simulink model "fw_pos_control"  (R2021a)
settings: Solver=FixedStepAuto  StartTime=0.0  StopTime=5  FixedStep=0.02  RelTol=1e-3
undefined symbols (not defined in the file): DiscIntNeverNeededParam, DT_DEFAULT, FW_AIRSPD_MAX, FW_AIRSPD_MIN, FW_L1_DAMPING, FW_L1_PERIOD, FW_L1_R_SLEW_MAX, FW_R_LIM, FW_T_CLMB_MAX, FW_T_HRATE_FF, FW_T_I_GAIN_PIT, FW_T_I_GAIN_THR, FW_T_PTCH_DAMP, FW_T_RLL2THR, FW_T_SEB_R_FF, FW_T_SINK_MAX, FW_T_SINK_MIN, FW_T_SPD_OMEGA, FW_T_STE_R_TC, FW_T_TAS_TC, FW_T_THR_DAMP, FW_T_VERT_ACC, FW_THR_CRUISE, FW_THR_MAX, FW_THR_MIN, FW_THR_SLEW_MAX, GRAVITY, magnitude
libraries: simulink x28, vrlib x3
(part 2 of 4)

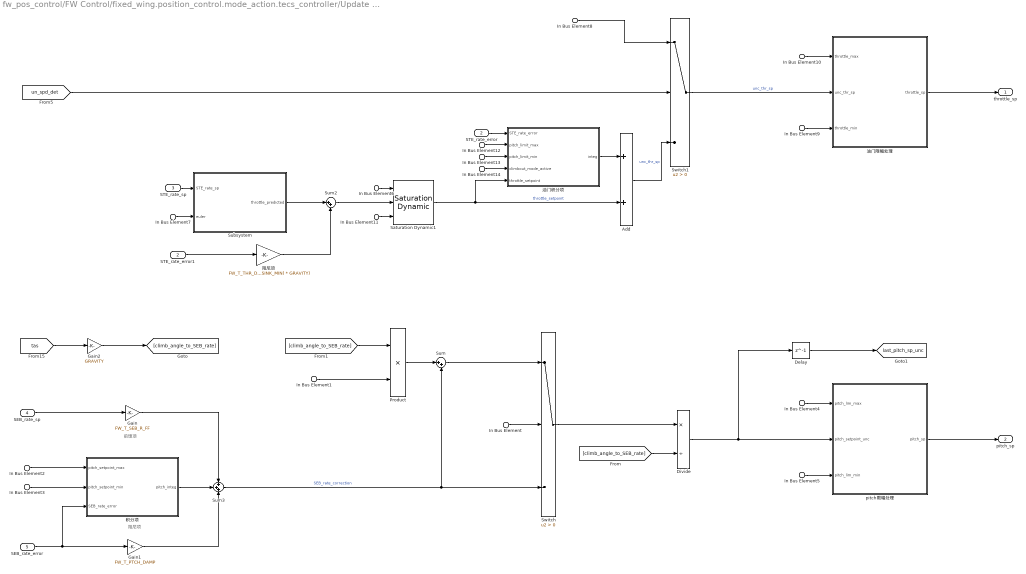
== system fw_pos_control/FW Control/fixed_wing.position_control.mode_action.tecs_controller/Update Throttle Setpoint and Pitch Setpoint ==
  note: 前馈项
  note: 阻尼项
  In Bus Element : Inport  PortName=tecs  Element=climb_out_setpoint
  In Bus Element14 : Inport  PortName=tecs  Element=climb_out_setpoint
  In Bus Element2 : Inport  PortName=tecs  Element=pitch_limit_max
  In Bus Element4 : Inport  PortName=tecs  Element=pitch_limit_max
  In Bus Element12 : Inport  PortName=tecs  Element=pitch_limit_max
  In Bus Element{1,3,5,13} (4 alike) : Inport  PortName=tecs  Element=pitch_limit_min
  In Bus Element11 : Inport  PortName=tecs  Element=throttle_min
  In Bus Element9 : Inport  PortName=tecs  Element=throttle_min
  In Bus Element10 : Inport  PortName=tecs  Element=throttle_max
  In Bus Element8 : Inport  PortName=tecs  Element=throttle_max
  In Bus Element6 : Inport  PortName=tecs  Element=throttle_max
  In Bus Element7 : Inport  PortName=tecs  Element=euler
  STE_rate_error : Inport  Port=2
  STE_rate_sp : Inport  Port=3
  SEB_rate_sp : Inport  Port=4
  SEB_rate_error : Inport  Port=5
  Add : Sum
  Delay : Delay  DelayLength=1
  Divide : Product  Inputs=*/
  Gain : Gain  Gain=FW_T_SEB_R_FF
      settings: AttributesFormatString=%<Gain>
  Gain1 : Gain  Gain=FW_T_PTCH_DAMP
      settings: AttributesFormatString=%<Gain>
  Gain2 : Gain  Gain=GRAVITY
      settings: AttributesFormatString=%<Gain>
  Product : Product
  STE_rate_error1 : InportShadow  Port=2
  Saturation Dynamic1 : simulink/Discontinuities/Saturation Dynamic  OutMin=[]  OutMax=[]  OutDataTypeStr=Inherit: Same as second input  OutDataType=fixdt(1, 16)  OutScaling=2^-10  DoSatur=off
  Subsystem : Subsystem
  Sum : Sum  Inputs=|++
  Sum2 : Sum  Inputs=|++
  Sum3 : Sum  Inputs=+++
  Switch : Switch  Criteria=u2 > Threshold
  Switch1 : Switch  Criteria=u2 > Threshold
  pitch限幅处理 : Subsystem
  油门积分项 : Subsystem
  油门限幅处理 : Subsystem
  积分项 : Subsystem
  阻尼项 : Gain  Gain=FW_T_THR_DAMP / ((FW_T_CLMB_MAX - FW_T_SINK_MIN) * GRAVITY)  OutDataTypeStr=single
      settings: AttributesFormatString=%<Gain>
  throttle_sp : Outport
  pitch_sp : Outport  Port=2
  tag scope: last_pitch_sp_unc=global
  wires:
  pitch限幅处理/1(pitch_sp) -> pitch_sp/1
  Divide/1 -> Delay/1, pitch限幅处理/2(pitch_setpoint_unc)
  SEB_rate_error/1 -> 积分项/3(SEB_rate_error), Gain1/1
  Delay/1 -> [last_pitch_sp_unc]
  积分项/1(pitch_integ) -> Sum3/2
  Gain/1 -> Sum3/1
  SEB_rate_sp/1 -> Gain/1
  Gain1/1 -> Sum3/3
  Sum3/1 -> Sum/2, Switch/3  "SEB_rate_correction"
  In Bus Element/1 -> Switch/2
  In Bus Element3/1 -> 积分项/2(pitch_setpoint_min)
  In Bus Element2/1 -> 积分项/1(pitch_setpoint_max)
  Switch/1 -> Divide/1
  Gain2/1 -> [climb_angle_to_SEB_rate]
  [tas] -> Gain2/1
  [climb_angle_to_SEB_rate] -> Divide/2
  [climb_angle_to_SEB_rate] -> Product/1
  In Bus Element1/1 -> Product/2
  Product/1 -> Sum/1
  Sum/1 -> Switch/1
  In Bus Element4/1 -> pitch限幅处理/1(pitch_lim_max)
  In Bus Element5/1 -> pitch限幅处理/3(pitch_lim_min)
  Saturation Dynamic1/1 -> 油门积分项/5(throttle_setpoint), Add/2  "throttle_setpoint"
  Subsystem/1(throttle_predicted) -> Sum2/1
  Switch1/1 -> 油门限幅处理/2(unc_thr_sp)  "unc_thr_sp"
  In Bus Element9/1 -> 油门限幅处理/3(throttle_min)
  Add/1 -> Switch1/3  "unc_thr_sp"
  In Bus Element6/1 -> Saturation Dynamic1/1
  In Bus Element8/1 -> Switch1/1
  阻尼项/1 -> Sum2/2
  [un_spd_det] -> Switch1/2
  In Bus Element10/1 -> 油门限幅处理/1(throttle_max)
  油门限幅处理/1(throttle_sp) -> throttle_sp/1
  STE_rate_error/1 -> 油门积分项/1(STE_rate_error)
  In Bus Element11/1 -> Saturation Dynamic1/3
  油门积分项/1(integ) -> Add/1
  Sum2/1 -> Saturation Dynamic1/2
  STE_rate_sp/1 -> Subsystem/1(STE_rate_sp)
  In Bus Element12/1 -> 油门积分项/2(pitch_limit_max)
  In Bus Element14/1 -> 油门积分项/4(climbout_mode_active)
  In Bus Element13/1 -> 油门积分项/3(pitch_limit_min)
  In Bus Element7/1 -> Subsystem/2(euler)
  STE_rate_error1/1 -> 阻尼项/1

== system fw_pos_control/FW Control/fixed_wing.position_control.mode_action.l1_navigate_loiter/Circle Mode/PD Terms ==
  note: $lateral\_accel\_sp\_circle\_pd = (xtrack\_err\_circle \times K\_crosstrack + xtrack\_vel\_circle \times K\_velocity);$
  xtrack_err_circle : Inport
  xtrack_vel_circle : Inport  Port=2
  circle_mode : Inport  Port=3
  AND : Logic  IconShape=distinctive  AllPortsSameDT=off  OutDataTypeStr=boolean
  Compare To Zero : simulink/Logic and Bit Operations/Compare To Zero  relop=<  OutDataTypeStr=boolean
  Gain1 : Gain  Gain=(2 * pi / FW_L1_PERIOD)^2
      settings: AttributesFormatString=%<Gain>
  Gain2 : Gain  Gain=(2 * pi / FW_L1_PERIOD)^2
      settings: AttributesFormatString=%<Gain>
  Gain3 : Gain  Gain=2 * FW_L1_DAMPING * (2 * pi / FW_L1_PERIOD)
      settings: AttributesFormatString=%<Gain>
  Gain5 : Gain  Gain=2 * FW_L1_DAMPING * (2 * pi / FW_L1_PERIOD)
      settings: AttributesFormatString=%<Gain>
  Saturation2 : Saturate  UpperLimit=0  LowerLimit=-inf
      settings: AttributesFormatString=[%<LowerLimit>,%<UpperLimit>]
  Sum1 : Sum  Inputs=|++
  Sum4 : Sum  Inputs=|++
  Switch2 : Switch  Criteria=u2 > Threshold
  xtrack_err_circle_1 : InportShadow
  xtrack_vel_circle_1 : InportShadow  Port=2
  lateral_accel_sp_circle_pd : Outport
  wires:
  xtrack_vel_circle_1/1 -> Gain5/1
  Saturation2/1 -> Switch2/1
  circle_mode/1 -> AND/2
  [tangent_vel] -> Compare To Zero/1
  Gain5/1 -> Sum4/2
  xtrack_err_circle/1 -> Gain2/1
  Compare To Zero/1 -> AND/1
  Gain1/1 -> Sum4/1
  Sum4/1 -> Switch2/3
  Gain3/1 -> Sum1/2
  xtrack_vel_circle/1 -> Gain3/1
  Sum1/1 -> Saturation2/1
  xtrack_err_circle_1/1 -> Gain1/1
  AND/1 -> Switch2/2
  Gain2/1 -> Sum1/1
  Switch2/1 -> lateral_accel_sp_circle_pd/1

== system fw_pos_control/FW Control/fixed_wing.position_control.mode_action.l1_navigate_loiter/Switch Lateral Accel Setpoint/If Action Subsystem ==
  lateral_accel_sp_center : Inport
  Action Port : ActionPort  ActionPortLabel=if(u1)
  Constant : Constant  Value=false
  circle_mode : Outport
  lateral_accel_sp : Outport  Port=2
  wires:
  Constant/1 -> circle_mode/1
  lateral_accel_sp_center/1 -> lateral_accel_sp/1

== system fw_pos_control/FW Control/fixed_wing.position_control.mode_action.l1_navigate_loiter/Switch Lateral Accel Setpoint/If Action Subsystem1 ==
  lateral_accel_sp_circle1 : Inport
  Action Port : ActionPort  ActionPortLabel=else
  Constant1 : Constant  Value=true
  lateral_accel_sp : Outport
  circle_mode : Outport  Port=2
  wires:
  lateral_accel_sp_circle1/1 -> lateral_accel_sp/1
  Constant1/1 -> circle_mode/1

== system fw_pos_control/FW Control/fixed_wing.position_control.mode_action.l1_navigate_loiter/Switch Lateral Accel Setpoint/Update Roll Setpoint ==
  att_sp_roll_body : Inport  PortDimensions=1
  lateral_accel : Inport  Port=2
  Compare To Zero : simulink/Logic and Bit Operations/Compare To Zero  relop=>  OutDataTypeStr=boolean
  Constant1 : Constant  Value=FW_L1_R_SLEW_MAX
      settings: AttributesFormatString=%<Value>
  Constant2 : Constant  Value=FW_L1_R_SLEW_MAX
      settings: AttributesFormatString=%<Value>
  Gain : Gain  Gain=1.0 / GRAVITY
      settings: AttributesFormatString=%<Gain>
  IsFinite1 : RelationalOperator  Operator=isFinite  OutDataTypeStr=boolean  RndMeth=Simplest
  Saturation : Saturate  UpperLimit=FW_R_LIM  LowerLimit=-FW_R_LIM
      settings: AttributesFormatString=[%<LowerLimit>,%<UpperLimit>]
  Saturation Dynamic : simulink/Discontinuities/Saturation Dynamic  OutMin=[]  OutMax=[]  OutDataTypeStr=Inherit: Same as second input  OutDataType=fixdt(1, 16)  OutScaling=2^-10  DoSatur=off
  Sum : Sum  Inputs=|++
  Sum1 : Sum  Inputs=-+|
  Switch1 : Switch  Criteria=u2 > Threshold
  Switch2 : Switch  Criteria=u2 > Threshold
  Weighted Sample Time : SampleTimeMath  TsampMathOp=*
  att_sp_roll_body_1 : InportShadow  PortDimensions=1
  att_sp_roll_body_2 : InportShadow  PortDimensions=1
  roll_sp : Outport
  wires:
  att_sp_roll_body/1 -> Sum/1
  Sum/1 -> Saturation Dynamic/1
  Weighted Sample Time/1 -> Sum/2, Sum1/1
  att_sp_roll_body_2/1 -> Switch2/3
  Saturation/1 -> IsFinite1/1, Switch2/1, Saturation Dynamic/2  "roll_new"
  Compare To Zero/1 -> Switch1/2
  Constant2/1 -> Compare To Zero/1
  Constant1/1 -> Weighted Sample Time/1
  Switch2/1 -> Switch1/3
  Sum1/1 -> Saturation Dynamic/3
  IsFinite1/1 -> Switch2/2
  att_sp_roll_body_1/1 -> Sum1/2
  Gain/1 -> Saturation/1
  Saturation Dynamic/1 -> Switch1/1
  Switch1/1 -> roll_sp/1
  lateral_accel/1 -> Gain/1

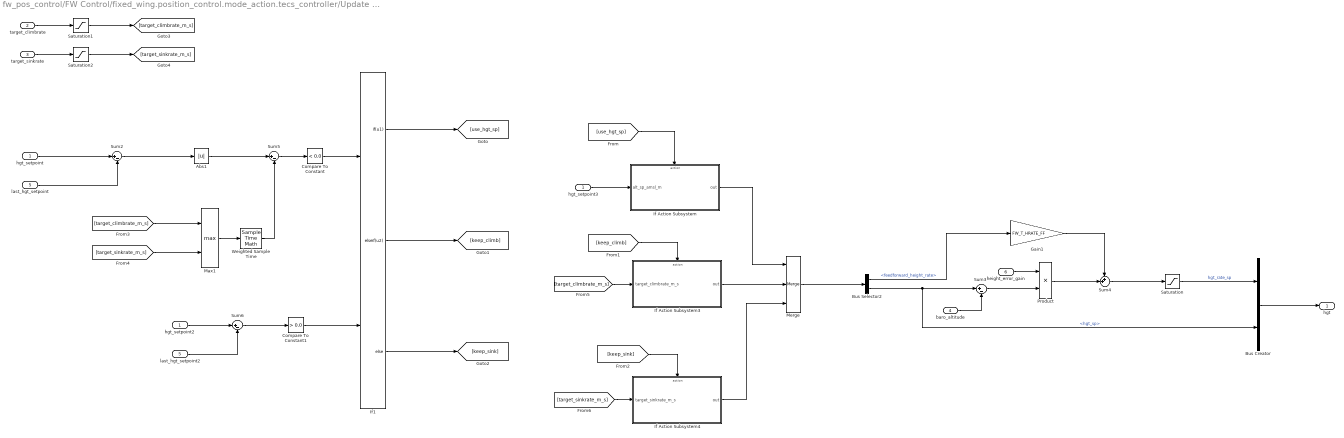
== system fw_pos_control/FW Control/fixed_wing.position_control.mode_action.tecs_controller/Update Height State and Height Setpoint State/Update Height Rate Setpoint ==
  hgt_setpoint : Inport
  target_climbrate : Inport  Port=2
  target_sinkrate : Inport  Port=3
  baro_altitude : Inport  Port=4
  last_hgt_setpoint : Inport  Port=5
  height_error_gain : Inport  Port=6
  Abs1 : Abs
  Bus Creator : BusCreator  Inputs=2
  Bus Selector2 : BusSelector  OutputSignals=feedforward_height_rate,hgt_sp
  Compare To Constant : simulink/Logic and Bit Operations/Compare To Constant  relop=<  const=0.0  OutDataTypeStr=boolean
  Compare To Constant1 : simulink/Logic and Bit Operations/Compare To Constant  relop=>  const=0.0  OutDataTypeStr=boolean
  Gain1 : Gain  Gain=FW_T_HRATE_FF
  If Action Subsystem : Subsystem  TreatAsAtomicUnit=on
  If Action Subsystem3 : Subsystem  TreatAsAtomicUnit=on
  If Action Subsystem4 : Subsystem  TreatAsAtomicUnit=on
  If1 : If  NumInputs=2  IfExpression=u1  ElseIfExpressions=u2
  Max1 : MinMax  Function=max  Inputs=2
  Merge : Merge  Inputs=3
  Product : Product
  Saturation : Saturate  UpperLimit=FW_T_CLMB_MAX  LowerLimit=-FW_T_SINK_MAX
      settings: AttributesFormatString=[%<LowerLimit>,%<UpperLimit>]
  Saturation1 : Saturate  UpperLimit=FW_T_CLMB_MAX  LowerLimit=-inf
      settings: AttributesFormatString=[%<LowerLimit>,%<UpperLimit>]
  Saturation2 : Saturate  UpperLimit=FW_T_SINK_MAX  LowerLimit=-inf
      settings: AttributesFormatString=[%<LowerLimit>,%<UpperLimit>]
  Sum{2..3,5..6} (4 alike) : Sum  Inputs=|+-
  Sum4 : Sum  Inputs=++|
  Weighted Sample Time : SampleTimeMath  TsampMathOp=*
  hgt_setpoint2 : InportShadow
  hgt_setpoint3 : InportShadow
  last_hgt_setpoint2 : InportShadow  Port=5
  hgt : Outport
  wires:
  hgt_setpoint3/1 -> If Action Subsystem/1(alt_sp_amsl_m)
  Merge/1 -> Bus Selector2/1
  If Action Subsystem/1(out) -> Merge/1
  If Action Subsystem3/1(out) -> Merge/2
  If Action Subsystem4/1(out) -> Merge/3
  Bus Selector2/2 -> Sum3/1, Bus Creator/2  "<hgt_sp>"
  Bus Selector2/1 -> Gain1/1  "<feedforward_height_rate>"
  Saturation/1 -> Bus Creator/1  "hgt_rate_sp"
  Sum4/1 -> Saturation/1
  Product/1 -> Sum4/2
  Gain1/1 -> Sum4/1
  Sum3/1 -> Product/2
  baro_altitude/1 -> Sum3/2
  target_climbrate/1 -> Saturation1/1
  target_sinkrate/1 -> Saturation2/1
  hgt_setpoint/1 -> Sum2/1
  last_hgt_setpoint/1 -> Sum2/2
  Max1/1 -> Weighted Sample Time/1
  Sum2/1 -> Abs1/1
  Abs1/1 -> Sum5/1
  Weighted Sample Time/1 -> Sum5/2
  Sum5/1 -> Compare To Constant/1
  last_hgt_setpoint2/1 -> Sum6/2
  hgt_setpoint2/1 -> Sum6/1
  Sum6/1 -> Compare To Constant1/1
  Compare To Constant/1 -> If1/1
  Compare To Constant1/1 -> If1/2
  If1/1 -> [use_hgt_sp]
  If1/3 -> [keep_sink]
  If1/2 -> [keep_climb]
  [use_hgt_sp] -> If Action Subsystem/Action
  [keep_climb] -> If Action Subsystem3/Action
  [keep_sink] -> If Action Subsystem4/Action
  Saturation2/1 -> [target_sinkrate_m_s]
  Saturation1/1 -> [target_climbrate_m_s]
  [target_climbrate_m_s] -> Max1/1
  [target_sinkrate_m_s] -> Max1/2
  [target_climbrate_m_s] -> If Action Subsystem3/1(target_climbrate_m_s)
  [target_sinkrate_m_s] -> If Action Subsystem4/1(target_sinkrate_m_s)
  height_error_gain/1 -> Product/1
  Bus Creator/1 -> hgt/1

== system fw_pos_control/FW Control/fixed_wing.position_control.mode_action.tecs_controller/Update Throttle Setpoint and Pitch Setpoint/Subsystem ==
  STE_rate_sp : Inport
  euler : Inport  Port=2
  1-D Lookup Table : Lookup_n-D  NumberOfTableDimensions=1  BreakpointsForDimension1=[0,FW_T_CLMB_MAX*GRAVITY]  Table=[FW_THR_CRUISE,FW_THR_MAX]  InternalRulePriority=Speed  RndMeth=Simplest  InputSameDT=on
  1-D Lookup Table1 : Lookup_n-D  NumberOfTableDimensions=1  BreakpointsForDimension1=[-FW_T_SINK_MIN*GRAVITY,0]  Table=[-FW_THR_MIN,FW_THR_CRUISE]  InternalRulePriority=Speed  RndMeth=Simplest  InputSameDT=on
  Constant1 : Constant  OutDataTypeStr=single
  Constant2 : Constant  Value=FW_T_CLMB_MAX * GRAVITY
      settings: AttributesFormatString=%<Value>
  Constant3 : Constant  Value=-FW_T_SINK_MIN * GRAVITY
      settings: AttributesFormatString=%<Value>
  Constant5 : Constant  OutDataTypeStr=single
  Cos1 : Trigonometry  Operator=cos
  Divide2 : Product  Inputs=*/
  Gain2 : Gain  Gain=FW_T_RLL2THR
  Saturation Dynamic : simulink/Discontinuities/Saturation Dynamic  OutMin=[]  OutMax=[]  OutDataTypeStr=Inherit: Same as second input  OutDataType=fixdt(1, 16)  OutScaling=2^-10  DoSatur=off
  Selector : Selector  InputPortWidth=3  IndexOptions=Index vector (dialog)  Indices=[1]  OutputSizes=1
  Sum : Sum  Inputs=|++
  Sum4 : Sum  Inputs=|+-
  Switch1 : Switch  Criteria=u2 > Threshold
  throttle_predicted : Outport
  wires:
  Sum4/1 -> Gain2/1
  Constant2/1 -> Saturation Dynamic/1
  Saturation Dynamic/1 -> 1-D Lookup Table1/1, 1-D Lookup Table/1, Switch1/2  "STE_rate_setpoint"
  Constant3/1 -> Saturation Dynamic/3
  Gain2/1 -> Sum/2
  Sum/1 -> Saturation Dynamic/2
  1-D Lookup Table1/1 -> Switch1/3
  Constant5/1 -> Sum4/2
  1-D Lookup Table/1 -> Switch1/1
  STE_rate_sp/1 -> Sum/1
  Switch1/1 -> throttle_predicted/1  "throttle_predicted"
  Cos1/1 -> Divide2/2
  Selector/1 -> Cos1/1
  Constant1/1 -> Divide2/1
  euler/1 -> Selector/1
  Divide2/1 -> Sum4/1

== system fw_pos_control/FW Control/fixed_wing.position_control.mode_action.tecs_controller/Update Throttle Setpoint and Pitch Setpoint/pitch限幅处理 ==
  pitch_lim_max : Inport
  pitch_setpoint_unc : Inport  Port=2
  pitch_lim_min : Inport  Port=3
  Constant : Constant  Value=FW_T_VERT_ACC
  Data Type Conversion : DataTypeConversion  OutDataTypeStr=single
  Delay1 : Delay  DelayLength=1
  Divide1 : Product  Inputs=*/
  Saturation Dynamic : simulink/Discontinuities/Saturation Dynamic  OutMin=[]  OutMax=[]  OutDataTypeStr=Inherit: Same as second input  OutDataType=fixdt(1, 16)  OutScaling=2^-10  DoSatur=off
  Saturation Dynamic1 : simulink/Discontinuities/Saturation Dynamic  OutMin=[]  OutMax=[]  OutDataTypeStr=Inherit: Same as second input  OutDataType=fixdt(1, 16)  OutScaling=2^-10  DoSatur=off
  Sum : Sum  Inputs=++|
  Sum1 : Sum  Inputs=-+|
  Weighted Sample Time : SampleTimeMath  TsampMathOp=*
  pitch_sp : Outport
  tag scope: last_pitch_sp=global
  wires:
  [tas] -> Divide1/2
  Delay1/1 -> [last_pitch_sp]
  Constant/1 -> Weighted Sample Time/1
  Sum/1 -> Saturation Dynamic1/1
  Saturation Dynamic1/1 -> Delay1/1, pitch_sp/1
  [last_pitch_sp] -> Sum1/2
  Sum1/1 -> Saturation Dynamic1/3
  pitch_lim_max/1 -> Saturation Dynamic/1
  Divide1/1 -> Sum1/1, Sum/1
  Weighted Sample Time/1 -> Data Type Conversion/1
  Saturation Dynamic/1 -> Saturation Dynamic1/2
  [last_pitch_sp] -> Sum/2
  pitch_lim_min/1 -> Saturation Dynamic/3
  pitch_setpoint_unc/1 -> Saturation Dynamic/2
  Data Type Conversion/1 -> Divide1/1

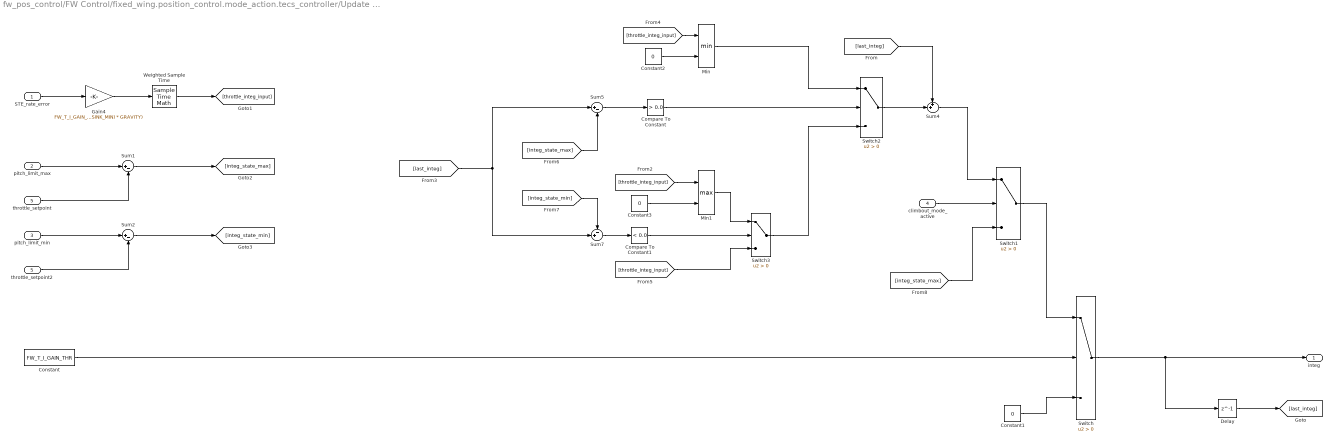
== system fw_pos_control/FW Control/fixed_wing.position_control.mode_action.tecs_controller/Update Throttle Setpoint and Pitch Setpoint/油门积分项 ==
  STE_rate_error : Inport
  pitch_limit_max : Inport  Port=2
  pitch_limit_min : Inport  Port=3
  climbout_mode_active : Inport  Port=4
  throttle_setpoint : Inport  Port=5
  Compare To Constant : simulink/Logic and Bit Operations/Compare To Constant  relop=>  const=0.0  OutDataTypeStr=boolean
  Compare To Constant1 : simulink/Logic and Bit Operations/Compare To Constant  relop=<  const=0.0  OutDataTypeStr=boolean
  Constant : Constant  Value=FW_T_I_GAIN_THR  OutDataTypeStr=single
  Constant1 : Constant  Value=0  OutDataTypeStr=single
  Constant2 : Constant  Value=0  OutDataTypeStr=single
  Constant3 : Constant  Value=0  OutDataTypeStr=single
  Delay : Delay  DelayLength=1
  Gain4 : Gain  Gain=FW_T_I_GAIN_THR / ((FW_T_CLMB_MAX - FW_T_SINK_MIN) * GRAVITY)  OutDataTypeStr=single
      settings: AttributesFormatString=%<Gain>
  Min : MinMax  Inputs=2
  Min1 : MinMax  Function=max  Inputs=2
  Sum1 : Sum  Inputs=|+-
  Sum2 : Sum  Inputs=|+-
  Sum4 : Sum  Inputs=++|
  Sum5 : Sum  Inputs=|+-
  Sum7 : Sum  Inputs=-+|
  Switch{,1..3} (4 alike) : Switch  Criteria=u2 > Threshold
  Weighted Sample Time : SampleTimeMath  TsampMathOp=*
  throttle_setpoint2 : InportShadow  Port=5
  integ : Outport
  wires:
  Sum5/1 -> Compare To Constant/1
  Gain4/1 -> Weighted Sample Time/1
  climbout_mode_active/1 -> Switch1/2
  Constant/1 -> Switch/2
  Switch1/1 -> Switch/1
  Switch/1 -> Delay/1, integ/1
  [integ_state_max] -> Switch1/3
  [last_integ] -> Sum4/1
  Sum4/1 -> Switch1/1
  STE_rate_error/1 -> Gain4/1
  Constant1/1 -> Switch/3
  Delay/1 -> [last_integ]
  [integ_state_max] -> Sum5/2
  [last_integ] -> Sum7/2, Sum5/1
  Sum7/1 -> Compare To Constant1/1
  Weighted Sample Time/1 -> [throttle_integ_input]
  Compare To Constant/1 -> Switch2/2
  [throttle_integ_input] -> Min/1
  Constant2/1 -> Min/2
  Min/1 -> Switch2/1
  Compare To Constant1/1 -> Switch3/2
  [throttle_integ_input] -> Min1/1
  Constant3/1 -> Min1/2
  Min1/1 -> Switch3/1
  Switch3/1 -> Switch2/3
  [throttle_integ_input] -> Switch3/3
  Switch2/1 -> Sum4/2
  throttle_setpoint/1 -> Sum1/2
  pitch_limit_max/1 -> Sum1/1
  Sum1/1 -> [integ_state_max]
  Sum2/1 -> [integ_state_min]
  throttle_setpoint2/1 -> Sum2/2
  pitch_limit_min/1 -> Sum2/1
  [integ_state_min] -> Sum7/1

== system fw_pos_control/FW Control/fixed_wing.position_control.mode_action.tecs_controller/Update Throttle Setpoint and Pitch Setpoint/油门限幅处理 ==
  throttle_max : Inport
  unc_thr_sp : Inport  Port=2
  throttle_min : Inport  Port=3
  Abs : Abs
  Constant1 : Constant  Value=FW_THR_SLEW_MAX  OutDataTypeStr=single
  Delay2 : Delay  DelayLength=1
  Gain : Gain  Gain=FW_THR_SLEW_MAX
      settings: AttributesFormatString=%<Gain>
  Saturation Dynamic : simulink/Discontinuities/Saturation Dynamic  OutMin=[]  OutMax=[]  OutDataTypeStr=Inherit: Same as second input  OutDataType=fixdt(1, 16)  OutScaling=2^-10  DoSatur=off
  Saturation Dynamic2 : simulink/Discontinuities/Saturation Dynamic  OutMin=[]  OutMax=[]  OutDataTypeStr=Inherit: Same as second input  OutDataType=fixdt(1, 16)  OutScaling=2^-10  DoSatur=off
  Sum : Sum  Inputs=|+-
  Sum1 : Sum  Inputs=++|
  Sum5 : Sum  Inputs=-+|
  Switch : Switch  Criteria=u2 > Threshold  Threshold=single(0.01)
  Weighted Sample Time : SampleTimeMath  TsampMathOp=*
  throttle_max1 : InportShadow
  throttle_min1 : InportShadow  Port=3
  unc_thr_sp1 : InportShadow  Port=2
  throttle_sp : Outport
  tag scope: last_thr_sp=global
  wires:
  [last_thr_sp] -> Sum5/2
  unc_thr_sp/1 -> Saturation Dynamic2/2
  [last_thr_sp] -> Sum1/1
  Abs/1 -> Switch/2
  Sum5/1 -> Saturation Dynamic2/3
  Sum1/1 -> Saturation Dynamic2/1
  Saturation Dynamic2/1 -> Switch/1
  Delay2/1 -> [last_thr_sp]
  Constant1/1 -> Abs/1
  unc_thr_sp1/1 -> Switch/3
  Switch/1 -> Saturation Dynamic/2
  throttle_max1/1 -> Saturation Dynamic/1
  throttle_min1/1 -> Saturation Dynamic/3
  Saturation Dynamic/1 -> Delay2/1, throttle_sp/1
  Gain/1 -> Weighted Sample Time/1
  throttle_max/1 -> Sum/1
  throttle_min/1 -> Sum/2
  Sum/1 -> Gain/1
  Weighted Sample Time/1 -> Sum1/2, Sum5/1

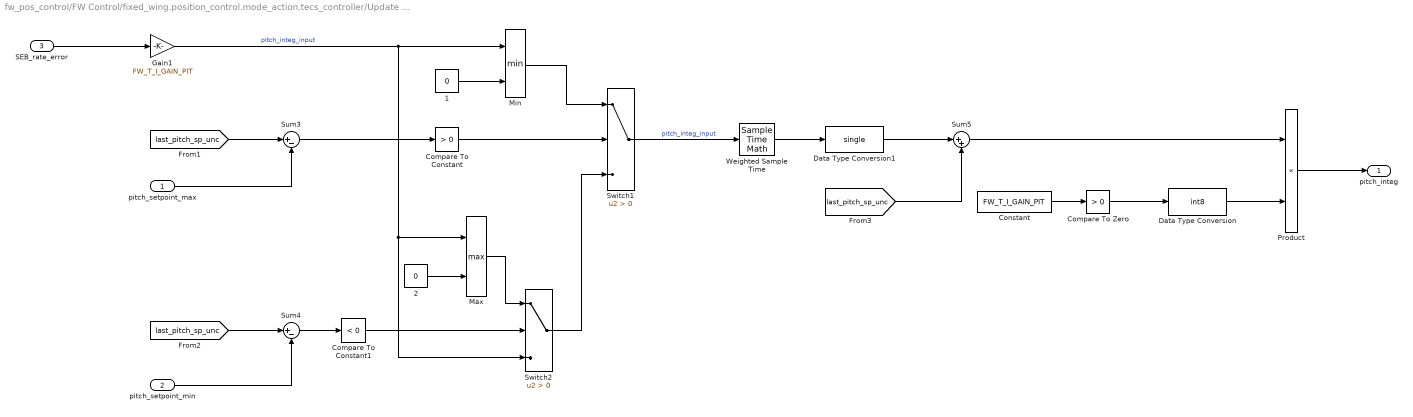
== system fw_pos_control/FW Control/fixed_wing.position_control.mode_action.tecs_controller/Update Throttle Setpoint and Pitch Setpoint/积分项 ==
  pitch_setpoint_max : Inport
  pitch_setpoint_min : Inport  Port=2
  SEB_rate_error : Inport  Port=3
  " 1" : Constant  Value=0  OutDataTypeStr=single
  " 2" : Constant  Value=0  OutDataTypeStr=single
  Compare To Constant : simulink/Logic and Bit Operations/Compare To Constant  relop=>  const=0  OutDataTypeStr=boolean
  Compare To Constant1 : simulink/Logic and Bit Operations/Compare To Constant  relop=<  const=0  OutDataTypeStr=boolean
  Compare To Zero : simulink/Logic and Bit Operations/Compare To Zero  relop=>  OutDataTypeStr=boolean
  Constant : Constant  Value=FW_T_I_GAIN_PIT
  Data Type Conversion : DataTypeConversion  OutDataTypeStr=int8
  Data Type Conversion1 : DataTypeConversion  OutDataTypeStr=single
  Gain1 : Gain  Gain=FW_T_I_GAIN_PIT
      settings: AttributesFormatString=%<Gain>
  Max : MinMax  Function=max  Inputs=2
  Min : MinMax  Inputs=2
  Product : Product
  Sum3 : Sum  Inputs=|+-
  Sum4 : Sum  Inputs=|+-
  Sum5 : Sum  Inputs=|++
  Switch1 : Switch  Criteria=u2 > Threshold
  Switch2 : Switch  Criteria=u2 > Threshold
  Weighted Sample Time : SampleTimeMath  TsampMathOp=*
  pitch_integ : Outport
  wires:
  Constant/1 -> Compare To Zero/1
  Product/1 -> pitch_integ/1
  Compare To Zero/1 -> Data Type Conversion/1
  Data Type Conversion/1 -> Product/2
  [last_pitch_sp_unc] -> Sum3/1
  pitch_setpoint_max/1 -> Sum3/2
  Gain1/1 -> Switch2/3, Max/1, Min/1  "pitch_integ_input"
  SEB_rate_error/1 -> Gain1/1
  Sum3/1 -> Compare To Constant/1
  [last_pitch_sp_unc] -> Sum4/1
  pitch_setpoint_min/1 -> Sum4/2
  Sum4/1 -> Compare To Constant1/1
  Compare To Constant/1 -> Switch1/2
  Compare To Constant1/1 -> Switch2/2
  Switch2/1 -> Switch1/3
  Min/1 -> Switch1/1
  " 1"/1 -> Min/2
  " 2"/1 -> Max/2
  Max/1 -> Switch2/1
  Switch1/1 -> Weighted Sample Time/1  "pitch_integ_input"
  Weighted Sample Time/1 -> Data Type Conversion1/1
  [last_pitch_sp_unc] -> Sum5/2
  Sum5/1 -> Product/1
  Data Type Conversion1/1 -> Sum5/1

== system fw_pos_control/FW Control/fixed_wing.position_control.mode_action.tecs_controller/Update Height State and Height Setpoint State/Update Height Rate Setpoint/If Action Subsystem ==
  alt_sp_amsl_m : Inport
  Action Port : ActionPort  ActionPortLabel=if(u1)
  Bus Creator1 : BusCreator  Inputs=2
  feedforward_height_rate : Constant  Value=0  OutDataTypeStr=single
  out : Outport
  wires:
  feedforward_height_rate/1 -> Bus Creator1/2  "feedforward_height_rate"
  alt_sp_amsl_m/1 -> Bus Creator1/1  "hgt_sp"
  Bus Creator1/1 -> out/1

== system fw_pos_control/FW Control/fixed_wing.position_control.mode_action.tecs_controller/Update Height State and Height Setpoint State/Update Height Rate Setpoint/If Action Subsystem3 ==
  target_climbrate_m_s : Inport
  Action Port : ActionPort  ActionPortLabel=elseif(u2)
  Bus Creator : BusCreator  Inputs=2
  Discrete-Time Integrator : DiscreteIntegrator  SampleTime=-1  ICPrevOutput=DiscIntNeverNeededParam  ICPrevScaledInput=DiscIntNeverNeededParam
  out : Outport
  wires:
  Bus Creator/1 -> out/1
  target_climbrate_m_s/1 -> Bus Creator/2, Discrete-Time Integrator/1  "feedforward_height_rate"
  Discrete-Time Integrator/1 -> Bus Creator/1  "hgt_sp"

== system fw_pos_control/FW Control/fixed_wing.position_control.mode_action.tecs_controller/Update Height State and Height Setpoint State/Update Height Rate Setpoint/If Action Subsystem4 ==
  target_sinkrate_m_s : Inport
  Action Port : ActionPort  ActionPortLabel=else
  Bus Creator : BusCreator  Inputs=2
  Discrete-Time Integrator : DiscreteIntegrator  SampleTime=-1  ICPrevOutput=DiscIntNeverNeededParam  ICPrevScaledInput=DiscIntNeverNeededParam
  Unary Minus1 : UnaryMinus
  out : Outport
  wires:
  Unary Minus1/1 -> Bus Creator/2, Discrete-Time Integrator/1  "feedforward_height_rate"
  target_sinkrate_m_s/1 -> Unary Minus1/1
  Bus Creator/1 -> out/1
  Discrete-Time Integrator/1 -> Bus Creator/1  "hgt_sp"

== matlab function fw_pos_control/FW Control/fixed_wing.position_control.mode_action.l1_navigate_loiter/MATLAB Function1 ==
  data: vector_3d output; origin input; vector_unit_3d output; target input; ground_speed_2d_ input; ground_speed_3d output; target_bearing output
% * Convert a 2D vector from WGS84 to planar coordinates.
% *
% This converts from latitude and longitude to planar
% coordinates with (0,0) being at the position of ref and
% returns a vector in meters towards wp.
%
% @param ref The reference position in WGS84 coordinates
% @param wp The point to convert to into the local coordinates, in WGS84 coordinates
% @return The vector in meters pointing from the reference position to the coordinates

function [vector_3d, vector_unit_3d, ground_speed_3d, target_bearing]  = get_local_planar_vector(origin, target, ground_speed_2d_)

CONSTANTS_RADIUS_OF_EARTH = 6371000;

% this is an approximation for small angles, proposed by [2]
x_angle = deg2rad(target(1) - origin(1));
y_angle = deg2rad(target(2) - origin(2));
x_origin_cos = cos(deg2rad(origin(1)));

vector_3d = [single(x_angle * CONSTANTS_RADIUS_OF_EARTH), single(y_angle * x_origin_cos * CONSTANTS_RADIUS_OF_EARTH)];

% prevent NaN when normalizing
if (norm(vector_3d) > single(eps))
    vector_unit_3d = [vector_3d / norm(vector_3d), single(0.0)];
else
    vector_unit_3d = [vector_3d, single(0.0)];
end

ground_speed_3d = [ground_speed_2d_, single(0.0)];

% 仅做输出使用
target_bearing = get_bearing_to_next_waypoint(target(1), target(2), origin(1), origin(2));

end
